simulink model "UD_model"  (R2021a)
settings: Solver=VariableStepAuto  StartTime=0.0  StopTime=10  MaxStep=1/60  RelTol=1e-3
PreLoadFcn:
  | load('parameters.mat');
undefined symbols (not defined in the file): coulomb_omega, Fc, gamma, Ku, omega0
libraries: vrlib x2
settings Model: EnablePacing=on  Creator=Patrick  LastModifiedBy=20191695
settings SolverCC: AlgebraicLoopSolver=TrustRegion
settings DataIOCC: ReturnWorkspaceOutputs=off
settings DebuggingCC: SFMachineParentedDataDiag=warning  ArithmeticOperatorsInVariantConditions=warning
settings SFSimCC: CustomCodeUndefinedFunction=UseInterfaceOnly

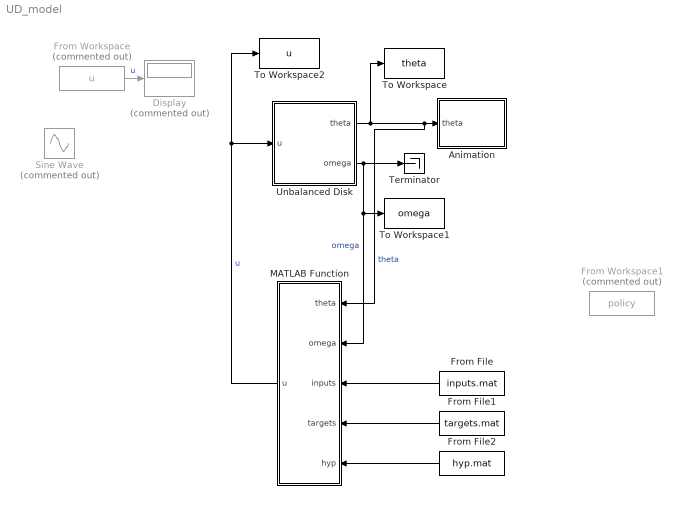
== system UD_model ==
  Animation : Subsystem
  Display : Display  Commented=on
  From Workspace : FromWorkspace  Commented=on  VariableName=u
  From Workspace1 : FromWorkspace  Commented=on  VariableName=policy
  From File : FromFile  FileName=inputs.mat  SampleTime=0
  From File1 : FromFile  FileName=targets.mat  SampleTime=0
  From File2 : FromFile  FileName=hyp.mat  SampleTime=0
  MATLAB Function : MATLAB Function  TreatAsAtomicUnit=on
  Sine Wave : Sin  Commented=on  Amplitude=3  Frequency=5  SampleTime=0
  Terminator : Terminator
  To Workspace : ToWorkspace  VariableName=theta  SampleTime=-1
  To Workspace1 : ToWorkspace  VariableName=omega  SaveFormat=Timeseries  SampleTime=-1
  To Workspace2 : ToWorkspace  VariableName=u  SaveFormat=Timeseries  SampleTime=-1
  Unbalanced Disk : Subsystem  mask{theta_0=0, omega_0=0}
      mask prompts: theta_0 "Initial condition theta"; omega_0 "Initial condition omega"
      mask DialogControl Param Prompt: Parameters
      mask Display: image('UnbalancedDisk.jpg');
  wires:
  MATLAB Function/1(u) -> To Workspace2/1, Unbalanced Disk/1(u)  "u"
  Unbalanced Disk/1(theta) -> To Workspace/1, Animation/1(theta), MATLAB Function/1(theta)  "theta"
  Unbalanced Disk/2(omega) -> MATLAB Function/2(omega), To Workspace1/1, Terminator/1  "omega"
  From Workspace/1 -> Display/1  "u"
  From File/1 -> MATLAB Function/3(inputs)
  From File1/1 -> MATLAB Function/4(targets)
  From File2/1 -> MATLAB Function/5(hyp)

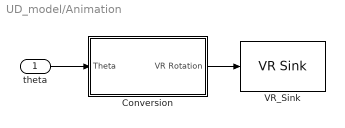
== system UD_model/Animation ==
  theta : Inport
  Conversion : Subsystem
  VR_Sink : vrlib/VR Sink  InstantiateOnLoad=on  SampleTime=-1  ViewEnable=on  RemoteChange=off  RemoteView=off  FieldsWritten=UD_Disc.rotation.4.1.1.double  WorldFileName=VR Model/UD_VR_World.wrl  AutoView=on  VideoDimensions=[]  AllowVariableSize=off  FigureProperties="{'Position', 'Name', 'Viewpoint', 'CameraBound', 'CameraDirection', 'CameraPosition', 'CameraUpVector', 'ZoomFactor', 'Antialiasing', 'Headlight', 'Lighting', 'NavPanel', 'Sound', 'StatusBar', 'Stereo3D', 'Stereo3DCameraOffset', 'Stereo3DHIT', 'ToolBar', 'Textures', 'Transparency', 'Triad', 'Wireframe', 'NavZones', 'NavMode', 'NavSpeed', 'CaptureFileFormat', 'CaptureFileName', 'Record2DCompressMethod', 'Record2DCompressQuality', 'Record2D', 'Record2DFileName', 'Record2DFPS'; [-1.7366000000000001e+03   3.1500000000000000e+02   5.7600000000000000e+02   3.5080000000000001e+02], '', 'Front View', 'on', [0.0000000000000000e+00   0.0000000000000000e+00  -1.0000000000000000e+00], [0.0000000000000000e+00   0.0000000000000000e+00  -5.0000000000000000e+00], [0.0000000000000000e+00   1.0000000000000000e+00   0.0000000000000000e+00], [1.0000000000000000e+00], 'on', 'on', 'off', 'halfbar', 'on', 'on', 'off', [1.0000000149011612e-01], [0.0000000000000000e+00], 'on', 'on', 'on', 'none', 'off', 'off', 'fly', 'normal', 'tif', '%f_anim_%n.tif', 'auto', [7.5000000000000000e+01], 'off', '%f_anim_%n.avi', 'auto'}"
  wires:
  theta/1 -> Conversion/1(Theta)
  Conversion/1(VR Rotation) -> VR_Sink/1

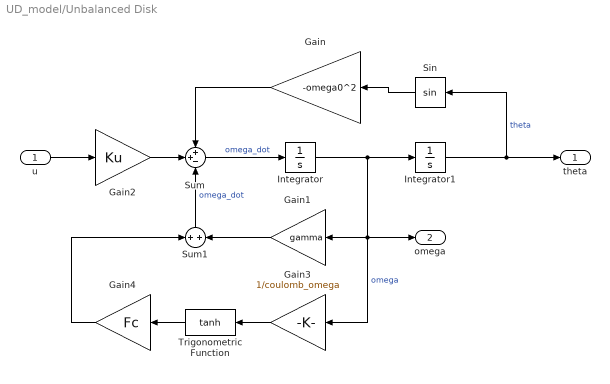
== system UD_model/Unbalanced Disk ==
  u : Inport
  Gain : Gain  Gain=-omega0^2
  Gain1 : Gain  Gain=gamma
  Gain2 : Gain  Gain=Ku
  Gain3 : Gain  Gain=1/coulomb_omega
  Gain4 : Gain  Gain=Fc
  Integrator : Integrator  InitialCondition=omega_0
  Integrator1 : Integrator  InitialCondition=theta_0
  Sin : Trigonometry
  Sum : Sum  Inputs=++-
  Sum1 : Sum
  Trigonometric Function : Trigonometry  Operator=tanh
  theta : Outport  VectorParamsAs1DForOutWhenUnconnected=off
  omega : Outport  Port=2  VectorParamsAs1DForOutWhenUnconnected=off
  wires:
  u/1 -> Gain2/1
  Sum/1 -> Integrator/1  "omega_dot"
  Sin/1 -> Gain/1
  Integrator/1 -> Gain3/1, omega/1, Gain1/1, Integrator1/1  "omega"
  Gain1/1 -> Sum1/2
  Gain2/1 -> Sum/2
  Integrator1/1 -> theta/1, Sin/1  "theta"
  Gain/1 -> Sum/1
  Gain3/1 -> Trigonometric Function/1
  Trigonometric Function/1 -> Gain4/1
  Gain4/1 -> Sum1/1
  Sum1/1 -> Sum/3  "omega_dot"

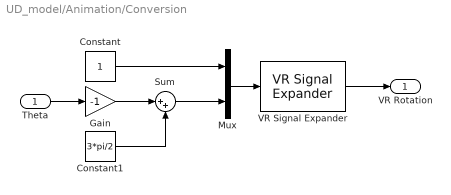
== system UD_model/Animation/Conversion ==
  Theta : Inport
  Constant : Constant
  Constant1 : Constant  Value=3*pi/2
  Gain : Gain  Gain=-1
  Mux : Mux  Inputs=2
  Sum : Sum  Inputs=|++
  VR Signal Expander : vrlib/VR Signal Expander  outwidth=4  outidx=[1 4]
  VR Rotation : Outport  VectorParamsAs1DForOutWhenUnconnected=off
  wires:
  Mux/1 -> VR Signal Expander/1
  Sum/1 -> Mux/2
  Gain/1 -> Sum/1
  Theta/1 -> Gain/1
  Constant1/1 -> Sum/2
  VR Signal Expander/1 -> VR Rotation/1
  Constant/1 -> Mux/1

== matlab function UD_model/MATLAB Function ==
  data: theta input; u output; omega input; inputs input; targets input; hyp input
function u = fcn(theta, omega, inputs, targets, hyp)

% henk = load("pendulum_23_H40.mat")
% henk = load('parameters.mat')

policy.fcn = @(policy,m,s)conCat(@congp,@gSat,policy,m,s);
policy.maxU = 3;
policy.p.inputs = inputs;
policy.p.targets = targets;
policy.p.hyp = hyp;

umax = 3;
poli = [1 3 4];

s = [omega sin(theta) cos(theta)]'
u = policy.fcn(policy,s,zeros(length(poli)));

% u(u>umax) = umax;                               % Clip input signal
% u(-umax>u) = -umax;
u = 2;
